simulink model "DC_2c_th"  (R2022b)
settings: Solver=VariableStepAuto  StartTime=0.0  StopTime=tEnd  MaxStep=1e-5  RelTol=1e-3
values from neighbouring files (symbols this model uses):
  A = [-R1/L1 -1/L1; 1/C1 0]    [DC_2_th.m]
  B = [1/L1; 0]    [DC_2_th.m]
  C = [0 1]    [DC_2_th.m]
  D = 0    [DC_2_th.m]
settings Model: Creator=alici  LastModifiedBy=alici

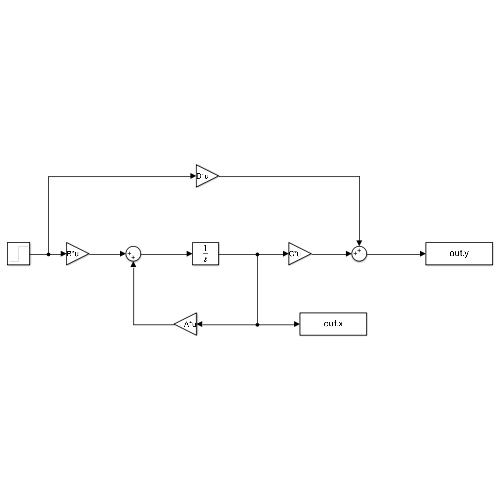
[thumbnail: Simulink's stored preview of the top-level diagram]
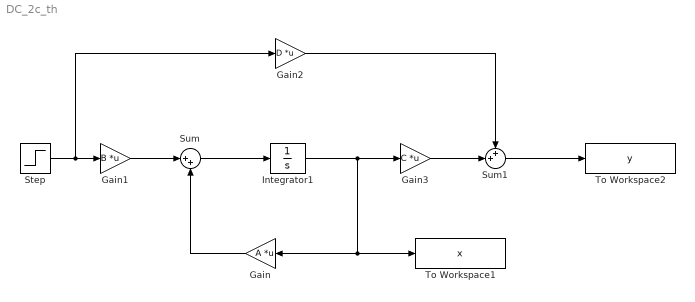
== system DC_2c_th ==
  Gain : Gain  Gain=A  Multiplication=Matrix(K*u)
  Gain1 : Gain  Gain=B  Multiplication=Matrix(K*u)
  Gain2 : Gain  Gain=D  Multiplication=Matrix(K*u)
  Gain3 : Gain  Gain=C  Multiplication=Matrix(K*u)
  Integrator1 : Integrator
  Step : Step  Time=0  SampleTime=0
  Sum : Sum  Inputs=|++
  Sum1 : Sum  Inputs=++|
  To Workspace1 : ToWorkspace  VariableName=x  SaveFormat=Timeseries  SampleTime=-1
  To Workspace2 : ToWorkspace  VariableName=y  SaveFormat=Timeseries  SampleTime=-1
  wires:
  Integrator1/1 -> Gain3/1, To Workspace1/1, Gain/1
  Step/1 -> Gain2/1, Gain1/1
  Gain1/1 -> Sum/1
  Gain/1 -> Sum/2
  Sum/1 -> Integrator1/1
  Gain2/1 -> Sum1/1
  Gain3/1 -> Sum1/2
  Sum1/1 -> To Workspace2/1
